simulink model "model1"  (R2021b)
settings: Solver=FixedStepAuto  StartTime=0.0  StopTime=350  FixedStep=0.01  RelTol=1e-3
values from neighbouring files (symbols this model uses):
  Cc = R2(2:end-1)    [calculateCc.m]    (also in demo2d.m = K2(2:end-1))
  k = 0    [Main.m]    (also in backupmain.m)
  kk = 0    [Main.m]    (also in backupmain.m)
  nbrpoints = A*[0 1]'    [Main.m]    (also in backupmain.m)
  theta0 = ThetaRef    [Main.m]    (also in backupmain.m)
  XYDpath = [Xpath;Ypath;DISTpath]    [Main.m]    (also in backupmain.m)
undefined symbols (not defined in the file or in its folder): s1, xR, y1, yR
libraries: simulink x2
settings Model: Creator=benal  LastModifiedBy=Ahmed Bellila

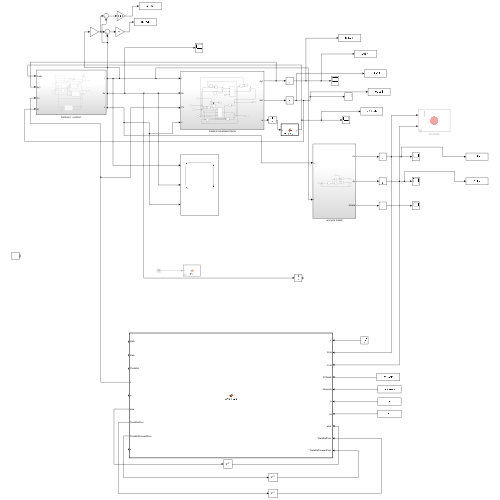
[thumbnail: Simulink's stored preview of the top-level diagram]
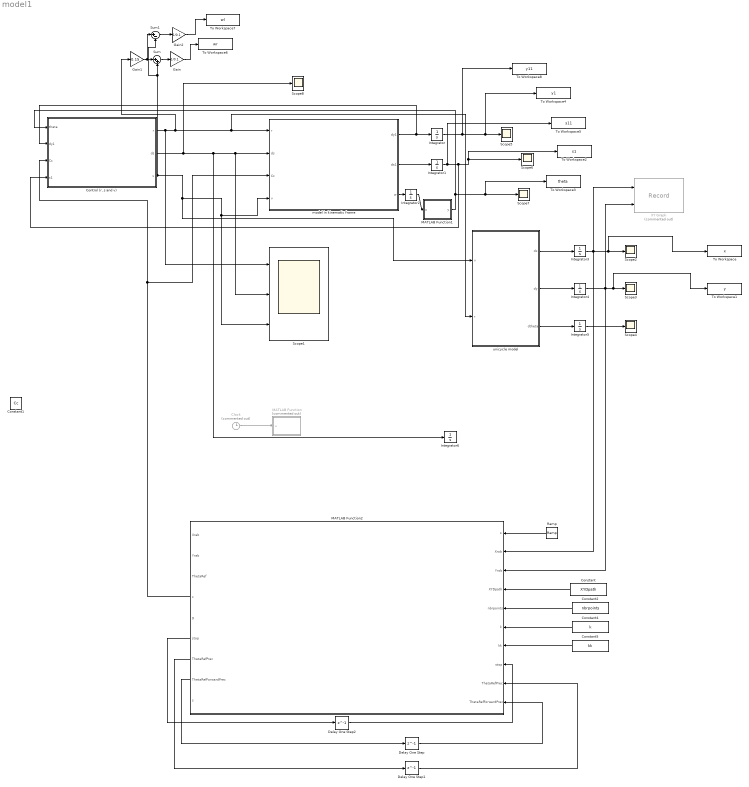
== system model1 ==
  Clock : Clock  Commented=on
  Constant : Constant  Value=XYDpath
  Constant1 : Constant  Value=Cc
  Constant2 : Constant  Value=nbrpoints
  Constant4 : Constant  Value=k
  Constant5 : Constant  Value=kk
  "Control (r, s and v)" : Subsystem
  Delay One Step : Delay  DelayLength=1
  Delay One Step1 : Delay  DelayLength=1
  Delay One Step2 : Delay  DelayLength=1
  Gain : Gain  Gain=1/0.1
  Gain1 : Gain  Gain=0.15
  Gain2 : Gain  Gain=1/0.1
  Integrator : Integrator  InitialCondition=y1
  Integrator1 : Integrator  InitialCondition=s1
  Integrator2 : Integrator  InitialCondition=theta0
  Integrator3 : Integrator  InitialCondition=xR
  Integrator4 : Integrator  InitialCondition=yR
  Integrator5 : Integrator  InitialCondition=theta0
  Integrator6 : Integrator  UpperSaturationLimit=XYDpath(3,2)  LowerSaturationLimit=-XYDpath(3,2)
  MATLAB Function : MATLAB Function  Commented=on  TreatAsAtomicUnit=on
  MATLAB Function1 : MATLAB Function  TreatAsAtomicUnit=on
  MATLAB Function2 : MATLAB Function  TreatAsAtomicUnit=on
  Ramp : simulink/Sources/Ramp  slope=2  start=0  InitialOutput=0
  Scope1 : Scope  NumInputPorts=3
  Scope{2..8} (7 alike) : Scope
  Sum : Sum  Inputs=|++
  Sum1 : Sum  Inputs=|+-
  To Workspace : ToWorkspace  VariableName=x  SampleTime=-1
  To Workspace1 : ToWorkspace  VariableName=y  SampleTime=-1
  To Workspace2 : ToWorkspace  VariableName=s1  SampleTime=-1
  To Workspace3 : ToWorkspace  VariableName=theta  SampleTime=-1
  To Workspace4 : ToWorkspace  VariableName=y1  SampleTime=-1
  To Workspace5 : ToWorkspace  VariableName=s11  SampleTime=-1
  To Workspace6 : ToWorkspace  VariableName=wr  SampleTime=-1
  To Workspace7 : ToWorkspace  VariableName=wl  SampleTime=-1
  To Workspace8 : ToWorkspace  VariableName=y11  SampleTime=-1
  XY Graph : Record  Commented=on  FileSettingsInternal="{\"entries\":[{\"content\":{\"excelSettings\":{\"content\":{},\"type\":\"Streamout.ExcelSettings\"}},\"type\":\"Streamout.FileSettingStorage\",\"uuid\":\"d9d5ad2c-9d1f-4f35-8b91-65b53c4d943b\"}],\"packageUris\":[\"http://schema.mathworks.com/mf0/streamout_blocks/R2020a\"],\"version\":\"1.0\"}"  Layout=[1 1]  SignalsInternal="{\"entries\":[{\"content\":{\"signals\":[{\"content\":{\"blockPath\":[\"model1/XY Graph\"],\"channel\":[],\"dimensions\":[1],\"domain\":\"model1/XY Graph\",\"lineColor\":\"#a2142f\",\"plots\":[1],\"port\":1,\"sid\":[],\"signalID\":107,\"signalName\":\"XY Graph:1\"},\"type\":\"RecordBlkView.Signal\",\"uuid\":\"66ddd082-d506-4df0-ad23-a651738e7c1e\"},{\"content\":{\"blockPath\":[\"model1/XY Graph\"],\"channel\":[],\"dimensions\":[1],\"domain\":\"model1/XY Graph\",\"lineColor\":\"#139fff\",\"plots\":[1],\"port\":2,\"sid\":[],\"signalID\":110,\"signalName\":\"XY Graph:2\"},\"type\":\"RecordBlkView.Signal\",\"uuid\":\"1661bbe3-8545-46ee-96ec-572f40a0cfb7\"}]},\"type\":\"RecordBlkView.InputSignals\",\"uuid\":\"26315ecb-f429-498c-a0d0-49db8a967ad3\"}],\"packageUris\":[\"http://schema.mathworks.com/mf0/streamout_blocks/R2020a\"],\"version\":\"1.0\"}"  VisualizationBindings="{\"xyplotplugin\":{\"info\":[{\"series\":[{\"bindingParametersList\":[{\"parameter\":\"X-Axis\",\"signalID\":107,\"signalName\":\"XY Graph:1\"},{\"parameter\":\"Y-Axis\",\"signalID\":110,\"signalName\":\"XY Graph:2\"}],\"seriesID\":65182}],\"subplotID\":1}]}}"  CompatibilityTag=XY  st=-1
  model in kinematic frame : Subsystem
  unicycle model : Subsystem
  wires:
  "Control (r, s and v)"/1(r) -> Scope1/1, Gain1/1, unicycle model/2(r), model in kinematic frame/1(r)
  "Control (r, s and v)"/3(v) -> unicycle model/1(v), Scope1/3, model in kinematic frame/4(v), Sum1/2, Sum/2
  model in kinematic frame/1(dy1) -> "Control (r, s and v)"/2(dy1), Integrator/1
  model in kinematic frame/3(w) -> Integrator2/1
  Integrator1/1 -> To Workspace5/1, Scope6/1, To Workspace2/1, "Control (r, s and v)"/4(s1)
  Integrator/1 -> To Workspace8/1, To Workspace4/1, Scope5/1
  MATLAB Function1/1(y) -> "Control (r, s and v)"/1(theta), To Workspace3/1, Scope7/1
  MATLAB Function2/4(c) -> model in kinematic frame/3(Cc), "Control (r, s and v)"/3(Cc)
  unicycle model/1(dx) -> Integrator3/1
  Integrator4/1 -> MATLAB Function2/3(Yrob), XY Graph/2, To Workspace1/1, Scope3/1
  unicycle model/2(dy) -> Integrator4/1
  unicycle model/3(dtheta) -> Integrator5/1
  Integrator5/1 -> Scope4/1
  Integrator3/1 -> MATLAB Function2/2(Xrob), XY Graph/1, To Workspace/1, Scope2/1
  model in kinematic frame/2(ds1) -> Integrator1/1
  Clock/1 -> MATLAB Function/1(u)
  Integrator2/1 -> MATLAB Function1/1(u)
  MATLAB Function2/8(ThetaRefForwardPrec) -> Delay One Step/1
  Constant4/1 -> MATLAB Function2/6(k)
  Constant5/1 -> MATLAB Function2/7(kk)
  Delay One Step/1 -> MATLAB Function2/10("ThetaRefForwardPrec ")
  MATLAB Function2/7(ThetaRefPrec) -> Delay One Step1/1
  Constant2/1 -> MATLAB Function2/5(nbrpoints)
  Constant/1 -> MATLAB Function2/4(XYDpath)
  Delay One Step1/1 -> MATLAB Function2/9("ThetaRefPrec ")
  MATLAB Function2/6(stop) -> Delay One Step2/1
  "Control (r, s and v)"/2(ds) -> Scope8/1, Integrator6/1, Scope1/2, model in kinematic frame/2(ds)
  Ramp/1 -> MATLAB Function2/1("s ")
  Delay One Step2/1 -> MATLAB Function2/8("stop ")
  Gain1/1 -> Sum1/1, Sum/1
  Sum/1 -> Gain/1
  Gain/1 -> To Workspace6/1
  Sum1/1 -> Gain2/1
  Gain2/1 -> To Workspace7/1

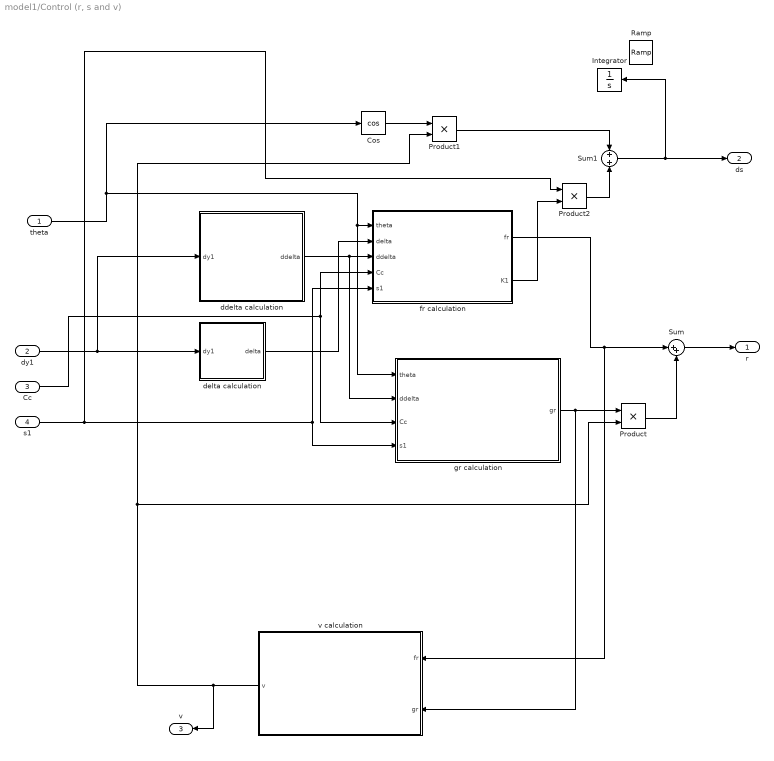
== system model1/Control (r, s and v) ==
  theta : Inport
  dy1 : Inport  Port=2
  Cc : Inport  Port=3
  s1 : Inport  Port=4
  Cos : Trigonometry  Operator=cos
  Integrator : Integrator  UpperSaturationLimit=XYDpath(3,2)  LowerSaturationLimit=-XYDpath(3,2)
  Product : Product
  Product1 : Product
  Product2 : Product
  Ramp : simulink/Sources/Ramp  slope=2  start=0  InitialOutput=0
  Sum : Sum  Inputs=|++
  Sum1 : Sum
  ddelta calculation : Subsystem
  delta calculation : Subsystem
  fr calculation : MATLAB Function  TreatAsAtomicUnit=on
  gr calculation : MATLAB Function  TreatAsAtomicUnit=on
  v calculation : MATLAB Function  TreatAsAtomicUnit=on
  r : Outport
  ds : Outport  Port=2
  v : Outport  Port=3
  wires:
  Cc/1 -> fr calculation/4(Cc), gr calculation/3(Cc)
  v calculation/1(v) -> v/1, Product1/2, Product/2
  s1/1 -> Product2/1, gr calculation/4(s1), fr calculation/5(s1)
  dy1/1 -> ddelta calculation/1(dy1), delta calculation/1(dy1)
  ddelta calculation/1(ddelta) -> gr calculation/2(ddelta), fr calculation/3(ddelta)
  Product/1 -> Sum/2
  theta/1 -> gr calculation/1(theta), fr calculation/1(theta), Cos/1
  Sum/1 -> r/1
  delta calculation/1(delta) -> fr calculation/2(delta)
  fr calculation/1(fr) -> v calculation/1(fr), Sum/1
  gr calculation/1(gr) -> v calculation/2(gr), Product/1
  Cos/1 -> Product1/1
  Product1/1 -> Sum1/1
  Product2/1 -> Sum1/2
  fr calculation/2(K1) -> Product2/2
  Sum1/1 -> Integrator/1, ds/1

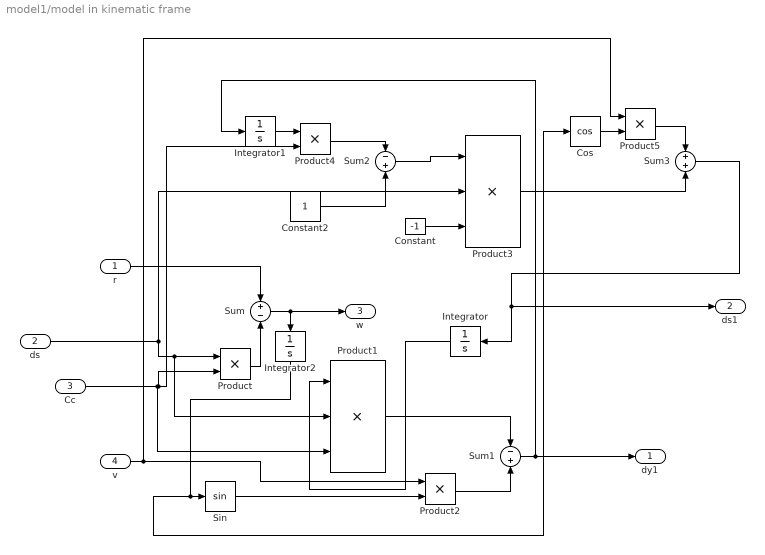
== system model1/model in kinematic frame ==
  r : Inport
  ds : Inport  Port=2
  Cc : Inport  Port=3
  v : Inport  Port=4
  Constant : Constant  Value=-1
  Constant2 : Constant
  Cos : Trigonometry  Operator=cos
  Integrator : Integrator  InitialCondition=s1
  Integrator1 : Integrator  InitialCondition=y1
  Integrator2 : Integrator  InitialCondition=theta0
  Product{,2,4..5} (4 alike) : Product
  Product1 : Product  Inputs=3
  Product3 : Product  Inputs=3
  Sin : Trigonometry
  Sum : Sum  Inputs=+-
  Sum1 : Sum  Inputs=-+
  Sum2 : Sum  Inputs=-+
  Sum3 : Sum
  dy1 : Outport
  ds1 : Outport  Port=2
  w : Outport  Port=3
  wires:
  Product/1 -> Sum/2
  v/1 -> Product2/1, Product5/1
  r/1 -> Sum/1
  Cc/1 -> Product1/3, Product4/2, Product/2
  Constant2/1 -> Sum2/2
  Integrator/1 -> Product1/1
  Cos/1 -> Product5/2
  Product5/1 -> Sum3/1
  Product3/1 -> Sum3/2
  Sum3/1 -> ds1/1, Integrator/1
  ds/1 -> Product3/2, Product1/2, Product/1
  Product1/1 -> Sum1/1
  Product4/1 -> Sum2/1
  Integrator2/1 -> Cos/1, Sin/1
  Sum/1 -> w/1, Integrator2/1
  Constant/1 -> Product3/3
  Product2/1 -> Sum1/2
  Sum2/1 -> Product3/1
  Sin/1 -> Product2/2
  Integrator1/1 -> Product4/1
  Sum1/1 -> Integrator1/1, dy1/1

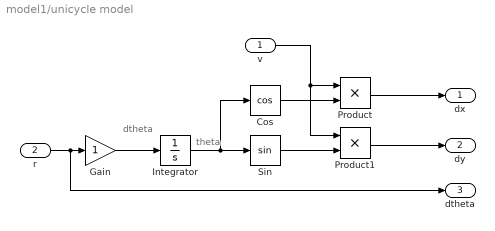
== system model1/unicycle model ==
  note: theta
  note: dtheta
  v : Inport
  r : Inport  Port=2
  Cos : Trigonometry  Operator=cos
  Gain : Gain
  Integrator : Integrator  InitialCondition=theta0
  Product : Product
  Product1 : Product
  Sin : Trigonometry
  dx : Outport
  dy : Outport  Port=2
  dtheta : Outport  Port=3
  wires:
  Integrator/1 -> Sin/1, Cos/1
  Product1/1 -> dy/1
  r/1 -> dtheta/1, Gain/1
  v/1 -> Product1/1, Product/1
  Sin/1 -> Product1/2
  Gain/1 -> Integrator/1
  Cos/1 -> Product/2
  Product/1 -> dx/1

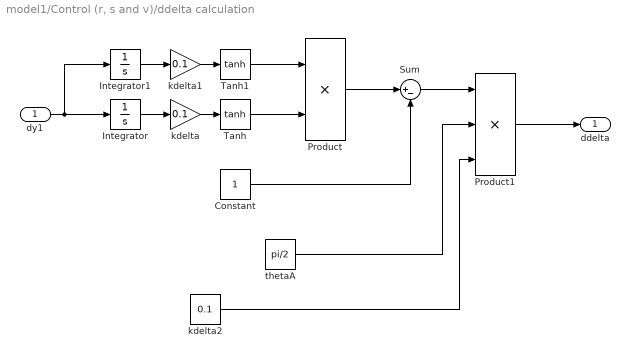
== system model1/Control (r, s and v)/ddelta calculation ==
  dy1 : Inport
  Constant : Constant
  Integrator : Integrator  InitialCondition=y1
  Integrator1 : Integrator  InitialCondition=y1
  Product : Product
  Product1 : Product  Inputs=3
  Sum : Sum  Inputs=|+-
  Tanh : Trigonometry  Operator=tanh
  Tanh1 : Trigonometry  Operator=tanh
  kdelta : Gain  Gain=0.1
  kdelta1 : Gain  Gain=0.1
  kdelta2 : Constant  Value=0.1
  thetaA : Constant  Value=pi/2
  ddelta : Outport
  wires:
  thetaA/1 -> Product1/2
  Tanh/1 -> Product/2
  kdelta1/1 -> Tanh1/1
  kdelta/1 -> Tanh/1
  kdelta2/1 -> Product1/3
  Integrator/1 -> kdelta/1
  dy1/1 -> Integrator1/1, Integrator/1
  Integrator1/1 -> kdelta1/1
  Product/1 -> Sum/1
  Tanh1/1 -> Product/1
  Product1/1 -> ddelta/1
  Constant/1 -> Sum/2
  Sum/1 -> Product1/1

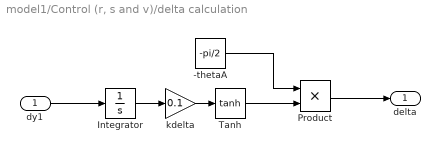
== system model1/Control (r, s and v)/delta calculation ==
  dy1 : Inport
  -thetaA : Constant  Value=-pi/2
  Integrator : Integrator  InitialCondition=y1
  Product : Product
  Tanh : Trigonometry  Operator=tanh
  kdelta : Gain  Gain=0.1
  delta : Outport
  wires:
  Integrator/1 -> kdelta/1
  Tanh/1 -> Product/2
  Product/1 -> delta/1
  dy1/1 -> Integrator/1
  -thetaA/1 -> Product/1
  kdelta/1 -> Tanh/1

== matlab function model1/Control (r, s and v)/gr calculation ==
  data: theta input; gr output; ddelta input; Cc input; s1 input
function gr = fcn(theta,ddelta,Cc,s1)

gr = Cc*cos(theta)*(1-s1*ddelta)+ddelta*sin(theta);

== matlab function model1/Control (r, s and v)/fr calculation ==
  data: theta input; fr output; delta input; ddelta input; Cc input; s1 input; K1 output
function [fr,K1] = fcn(theta,delta,ddelta,Cc,s1)
k1 = 1;
k2 = 1;

K1 = k1/(1+(s1*Cc*(1-s1*ddelta))^2);

fr = -k2*tanh(theta-delta)+K1*s1*Cc*(1-s1*ddelta);

== matlab function model1/Control (r, s and v)/v calculation ==
  data: fr input; v output; gr input
function v = fcn(fr,gr)
wmax = 2*pi;
R = 0.1;
L = 0.15;
vmax = (R*wmax-L*abs(fr))/(1+L*abs(gr));
v = (R*wmax-L*(1/4+fr^2))/(1+L*(1/4+gr^2));
v = min(v,vmax);

== matlab function model1/MATLAB Function ==
  data: u input
function  fcn(u)
    coder.extrinsic('bdroot')
    coder.extrinsic('set_param')
    if rem(u,0.1) == 0 && u ~= 0
        set_param(bdroot,'SimulationCommand','pause')
    end
end

== matlab function model1/MATLAB Function1 ==
  data: u input; y output
function y = wrapangle( u)
y = wrapToPi(u);

== matlab function model1/MATLAB Function2 ==
  data: s input; Xrab output; Xrob input; Yrob input; Yrab output; ThetaRef output; c output; g output; stop output; XYDpath input; nbrpoints input; k input; kk input; stop input; ThetaRefPrec output; ThetaRefForwardPrec output; ThetaRefPrec input; ThetaRefForwardPrec input; s output
function [Xrab,Yrab,ThetaRef,c,g,stop,ThetaRefPrec,ThetaRefForwardPrec,s]=SplinePath(s,Xrob,Yrob,XYDpath,nbrpoints,k,kk,stop,ThetaRefPrec,ThetaRefForwardPrec)


%test on s to locate the surrounding path points
i=2;
s = abs(s);

while(XYDpath(3,i)<=s && stop ~= 1)
    i=i+1;
    if (i>nbrpoints-100)
        disp('end of path reached')
        stop=1;
    end
end



%the surrounding points are X,Y(i-1) and X,Y(i)
%interpolation of the rabbit position



Xrab=XYDpath(1,i-1) + (XYDpath(1,i) - XYDpath(1,i-1))*(s - XYDpath(3,i-1))/(XYDpath(3,i) - XYDpath(3,i-1));
Yrab=XYDpath(2,i-1) + (XYDpath(2,i) - XYDpath(2,i-1))*(s - XYDpath(3,i-1))/(XYDpath(3,i) - XYDpath(3,i-1));

%%estimation of the rabbit global heading

%Counter on ThetaRef
ThetaReftest = atan2((XYDpath(2,i) - XYDpath(2,i-1)) , (XYDpath(1,i) - XYDpath(1,i-1)));
if (ThetaReftest - ThetaRefPrec > 1)
    k=k-1
    disp('k=k-1');
end
if (ThetaReftest - ThetaRefPrec < -1)
    k=k+1
    disp('k=k+1');
end
ThetaRef = ThetaReftest+2*k*pi;
ThetaRefPrec=ThetaReftest;

%Counter on ThetaRefForward
ThetaReftestForward = atan2((XYDpath(2,i+1) - XYDpath(2,i)) , (XYDpath(1,i+1) - XYDpath(1,i)));
if (ThetaReftestForward - ThetaRefForwardPrec > 1)
    kk=kk-1;
end
if (ThetaReftestForward - ThetaRefForwardPrec < -1)
    kk=kk+1;
end
ThetaRefForward = ThetaReftestForward+2*kk*pi;
ThetaRefForwardPrec=ThetaReftestForward;

c =(ThetaRefForward - ThetaRef)/(XYDpath(3,i+1) - XYDpath(3,i-1));
%c = 0;
g = 0;
%c = 0;
s1=-cos(ThetaRef)*(Xrab-Xrob)-sin(ThetaRef)*(Yrab-Yrob);
y1=sin(ThetaRef)*(Xrab-Xrob)-cos(ThetaRef)*(Yrab-Yrob);
